simulink model "pendulum_on_a_cart_ctrld"  (R2021a)
settings: Solver=daessc  StartTime=0.0  StopTime=simlength  RelTol=1e-3
undefined symbols (not defined in the file): Ad, Aled, Bd, Bled, C, Cle, g, Ked, Ld, Lled, tc, ts
libraries: nesl_utility x14, fl_lib x8, pendulum_on_a_cart_lib x2
settings Model: SimulationMode=accelerator  Creator=dbagn  LastModifiedBy=dabagnara
settings SolverCC: AlgebraicLoopSolver=TrustRegion
settings DataIOCC: ReturnWorkspaceOutputs=off
settings DebuggingCC: SFMachineParentedDataDiag=warning

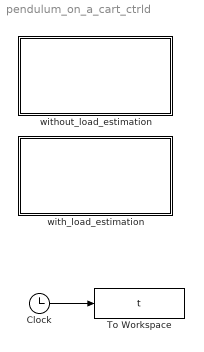
== system pendulum_on_a_cart_ctrld ==
  Clock : Clock
  To Workspace : ToWorkspace  VariableName=t  SampleTime=tc
      settings: MaxDataPoints=Nc
  with_load_estimation : Subsystem
  without_load_estimation : Subsystem
  wires:
  Clock/1 -> To Workspace/1

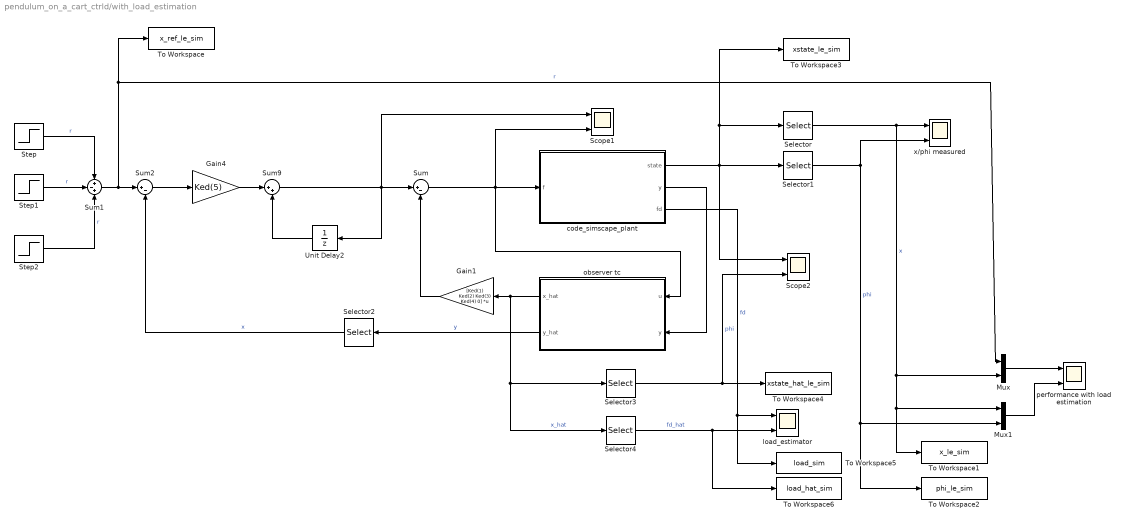
== system pendulum_on_a_cart_ctrld/with_load_estimation ==
  Gain1 : Gain  Gain=[Ked(1) Ked(2) Ked(3) Ked(4) 0]  Multiplication=Matrix(K*u)
  Gain4 : Gain  Gain=Ked(5)
  Mux : Mux  Inputs=2
  Mux1 : Mux  Inputs=2
  Scope1 : Scope  NumInputPorts=2
  Scope2 : Scope  NumInputPorts=2
  Selector : Selector  InputPortWidth=4  IndexOptions=Index vector (dialog)  Indices=1  OutputSizes=1
  Selector1 : Selector  InputPortWidth=4  IndexOptions=Index vector (dialog)  Indices=3  OutputSizes=1
  Selector2 : Selector  InputPortWidth=2  IndexOptions=Index vector (dialog)  Indices=1  OutputSizes=1
  Selector3 : Selector  InputPortWidth=5  IndexOptions=Index vector (dialog)  Indices=[1 2 3 4]  OutputSizes=1
  Selector4 : Selector  InputPortWidth=5  IndexOptions=Index vector (dialog)  Indices=5  OutputSizes=1
  Step : Step  SampleTime=0
  Step1 : Step  Time=8  After=2  SampleTime=0
  Step2 : Step  Time=25  SampleTime=0
  Sum : Sum  Inputs=|+-
  Sum1 : Sum  Inputs=+-+
  Sum2 : Sum  Inputs=|+-
  Sum9 : Sum  Inputs=|++
  To Workspace : ToWorkspace  VariableName=x_ref_le_sim  SampleTime=tc
      settings: MaxDataPoints=Nc
  To Workspace1 : ToWorkspace  VariableName=x_le_sim  SampleTime=tc
      settings: MaxDataPoints=Nc
  To Workspace2 : ToWorkspace  VariableName=phi_le_sim  SampleTime=tc
      settings: MaxDataPoints=Nc
  To Workspace3 : ToWorkspace  VariableName=xstate_le_sim  SampleTime=tc
      settings: MaxDataPoints=Nc
  To Workspace4 : ToWorkspace  VariableName=xstate_hat_le_sim  SampleTime=tc
      settings: MaxDataPoints=Nc
  To Workspace5 : ToWorkspace  VariableName=load_sim  SampleTime=tc
      settings: MaxDataPoints=Nc
  To Workspace6 : ToWorkspace  VariableName=load_hat_sim  SampleTime=tc
      settings: MaxDataPoints=Nc
  Unit Delay2 : UnitDelay  SampleTime=ts  HasFrameUpgradeWarning=on
  "code_simscape_plant " : Subsystem
  load_estimator : Scope  NumInputPorts=2
  observer tc : Subsystem
  performance with load estimation : Scope  NumInputPorts=2
  x/phi measured : Scope  NumInputPorts=2
  wires:
  Sum1/1 -> To Workspace/1, Mux/1, Sum2/1  "r"
  Sum2/1 -> Gain4/1
  Step1/1 -> Sum1/2  "r"
  Step/1 -> Sum1/1  "r"
  Gain4/1 -> Sum9/1
  observer tc/2(y_hat) -> Selector2/1  "y"
  Selector1/1 -> To Workspace2/1, Mux1/2, x/phi measured/2  "phi"
  "code_simscape_plant "/1(state) -> Scope2/1, Selector1/1, To Workspace3/1, Selector/1
  observer tc/1(x_hat) -> Gain1/1, Selector3/1, Selector4/1  "x_hat"
  Sum9/1 -> Scope1/1, Sum/1, Unit Delay2/1
  "code_simscape_plant "/2(y) -> observer tc/2(y)
  Selector2/1 -> Sum2/2  "x"
  Gain1/1 -> Sum/2
  Unit Delay2/1 -> Sum9/2
  Selector3/1 -> To Workspace4/1, Scope2/2  "phi"
  "code_simscape_plant "/3(fd) -> To Workspace5/1, load_estimator/1  "fd"
  Selector4/1 -> To Workspace6/1, load_estimator/2  "fd_hat"
  Step2/1 -> Sum1/3  "r"
  Mux1/1 -> performance with load estimation/2
  Mux/1 -> performance with load estimation/1
  Selector/1 -> To Workspace1/1, Mux1/1, Mux/2, x/phi measured/1  "x"
  Sum/1 -> observer tc/1(u), Scope1/2, "code_simscape_plant "/1(f)

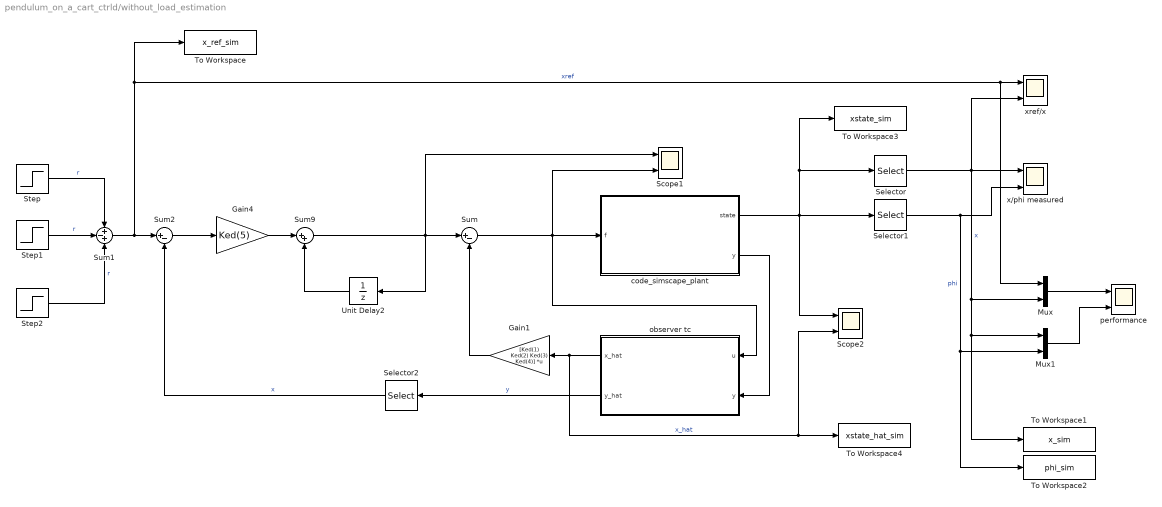
== system pendulum_on_a_cart_ctrld/without_load_estimation ==
  Gain1 : Gain  Gain=[Ked(1) Ked(2) Ked(3) Ked(4)]  Multiplication=Matrix(K*u)
  Gain4 : Gain  Gain=Ked(5)
  Mux : Mux  Inputs=2
  Mux1 : Mux  Inputs=2
  Scope1 : Scope  NumInputPorts=2
  Scope2 : Scope  NumInputPorts=2
  Selector : Selector  InputPortWidth=4  IndexOptions=Index vector (dialog)  Indices=1  OutputSizes=1
  Selector1 : Selector  InputPortWidth=4  IndexOptions=Index vector (dialog)  Indices=3  OutputSizes=1
  Selector2 : Selector  InputPortWidth=2  IndexOptions=Index vector (dialog)  Indices=1  OutputSizes=1
  Step : Step  SampleTime=0
  Step1 : Step  Time=8  After=2  SampleTime=0
  Step2 : Step  Time=25  SampleTime=0
  Sum : Sum  Inputs=|+-
  Sum1 : Sum  Inputs=+-+
  Sum2 : Sum  Inputs=|+-
  Sum9 : Sum  Inputs=|++
  To Workspace : ToWorkspace  VariableName=x_ref_sim  SampleTime=tc
      settings: MaxDataPoints=Nc
  To Workspace1 : ToWorkspace  VariableName=x_sim  SampleTime=tc
      settings: MaxDataPoints=Nc
  To Workspace2 : ToWorkspace  VariableName=phi_sim  SampleTime=tc
      settings: MaxDataPoints=Nc
  To Workspace3 : ToWorkspace  VariableName=xstate_sim  SampleTime=tc
      settings: MaxDataPoints=Nc
  To Workspace4 : ToWorkspace  VariableName=xstate_hat_sim  SampleTime=tc
      settings: MaxDataPoints=Nc
  Unit Delay2 : UnitDelay  SampleTime=ts  HasFrameUpgradeWarning=on
  "code_simscape_plant " : Subsystem
  observer tc : Subsystem
  performance : Scope  NumInputPorts=2
  x/phi measured : Scope  NumInputPorts=2
  xref/x : Scope  NumInputPorts=2
  wires:
  Unit Delay2/1 -> Sum9/2
  Gain1/1 -> Sum/2
  Selector2/1 -> Sum2/2  "x"
  Sum/1 -> "code_simscape_plant "/1(f), Scope1/2, observer tc/1(u)
  Selector/1 -> To Workspace1/1, Mux1/1, Mux/2, x/phi measured/1, xref/x/2  "x"
  "code_simscape_plant "/2(y) -> observer tc/2(y)
  Sum9/1 -> Unit Delay2/1, Sum/1, Scope1/1
  observer tc/1(x_hat) -> Scope2/2, To Workspace4/1, Gain1/1  "x_hat"
  "code_simscape_plant "/1(state) -> To Workspace3/1, Selector/1, Scope2/1, Selector1/1
  Selector1/1 -> To Workspace2/1, Mux1/2, x/phi measured/2  "phi"
  observer tc/2(y_hat) -> Selector2/1  "y"
  Gain4/1 -> Sum9/1
  Sum2/1 -> Gain4/1
  Sum1/1 -> To Workspace/1, Mux/1, xref/x/1, Sum2/1  "xref"
  Step/1 -> Sum1/1  "r"
  Step2/1 -> Sum1/3  "r"
  Step1/1 -> Sum1/2  "r"
  Mux/1 -> performance/1
  Mux1/1 -> performance/2

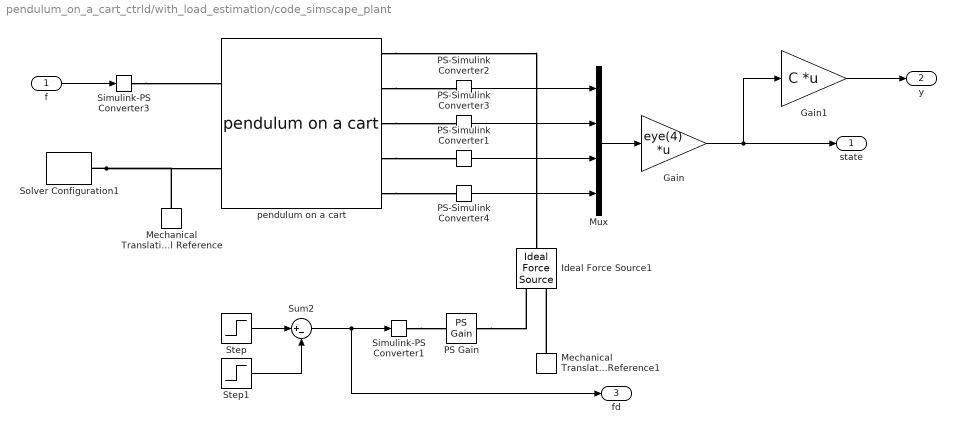
== system pendulum_on_a_cart_ctrld/with_load_estimation/code_simscape_plant  ==
  f : Inport
  Gain : Gain  Gain=eye(4)  Multiplication=Matrix(K*u)
  Gain1 : Gain  Gain=C  Multiplication=Matrix(K*u)
  Ideal Force Source1 : fl_lib/Mechanical/Mechanical Sources/Ideal Force Source
  Mechanical Translational Reference : fl_lib/Mechanical/Translational Elements/Mechanical Translational Reference
  Mechanical Translational Reference1 : fl_lib/Mechanical/Translational Elements/Mechanical Translational Reference
  Mux : Mux
  PS Gain : fl_lib/Physical Signals/Functions/PS Gain  gain=-1
  PS-Simulink Converter1 : nesl_utility/PS-Simulink Converter  PhysicalDomain=network_engine_domain  SubClassName=ps_output  LeftPortType=input  RightPortType=output  PseudoPeriodic=off  Frequencies=[]  Unit=rad  AffineConversion=on
      settings: SourceProductBaseCode=PW,SS
  PS-Simulink Converter2 : nesl_utility/PS-Simulink Converter  PhysicalDomain=network_engine_domain  SubClassName=ps_output  LeftPortType=input  RightPortType=output  PseudoPeriodic=off  Frequencies=[]  Unit=m  AffineConversion=on
      settings: SourceProductBaseCode=PW,SS
  PS-Simulink Converter3 : nesl_utility/PS-Simulink Converter  PhysicalDomain=network_engine_domain  SubClassName=ps_output  LeftPortType=input  RightPortType=output  PseudoPeriodic=off  Frequencies=[]  Unit=m/s  AffineConversion=on
      settings: SourceProductBaseCode=PW,SS
  PS-Simulink Converter4 : nesl_utility/PS-Simulink Converter  PhysicalDomain=network_engine_domain  SubClassName=ps_output  LeftPortType=input  RightPortType=output  PseudoPeriodic=off  Frequencies=[]  Unit=rad/s  AffineConversion=on
      settings: SourceProductBaseCode=PW,SS
  Simulink-PS Converter1 : nesl_utility/Simulink-PS Converter  PhysicalDomain=network_engine_domain  SubClassName=ps_input  LeftPortType=input  RightPortType=output  PseudoPeriodic=off  Frequencies=[]  NoiseDistribution=none  NoiseParameters=[]  Unit=N  AffineConversion=off  FilteringAndDerivatives=provide  SimscapeFilterOrder=1  InputFilterTimeConstant=0.001  UdotUserProvided=0
      settings: SourceProductBaseCode=PW,SS
  Simulink-PS Converter3 : nesl_utility/Simulink-PS Converter  PhysicalDomain=network_engine_domain  SubClassName=ps_input  LeftPortType=input  RightPortType=output  PseudoPeriodic=off  Frequencies=[]  NoiseDistribution=none  NoiseParameters=[]  Unit=N  AffineConversion=off  FilteringAndDerivatives=provide  SimscapeFilterOrder=1  InputFilterTimeConstant=0.001  UdotUserProvided=0
      settings: SourceProductBaseCode=PW,SS
  Solver Configuration1 : nesl_utility/Solver Configuration  PhysicalDomain=network_engine_domain  SubClassName=solver  LeftPortType=input  RightPortType=generic  Tones=[]  Harmonics=[]  SimulateNoise=off  Profile=off  UseLocalSampling=off  EnableSwitchedLinearOptims=on  FrequencyDomain=off  UseCCode=off  RelTol=0.001  AbsTol=1e-06  MinStep=1e-09  ToWorkspace=off  RevertToSquareIcSolve=off  NumHomotopyIterations=100  PhasorMode=off  PhasorModeNumHarmonics=1  DoDC=on  ResidualTolerance=1e-09  UseLocalSolver=off  LocalSolverChoice=NE_BACKWARD_EULER_ADVANCER  LocalSolverSampleTime=ts  DoFixedCost=off  MaxNonlinIter=3  MaxModeIter=2  ComputeImpulses=off  ImpulseIterations=2  LinearAlgebra=auto  EquationFormulation=NE_TIME_EF  DelaysMemoryBudget=1024  AutomaticFiltering=on  FilteringTimeConstant=0.001  PartitionStorageMethod=AS_NEEDED  PartitionMemoryBudget=1024  PartitionMethod=ROBUST
      settings: SourceProductBaseCode=PW,SS
  Step : Step  Time=17.5  After=1000  SampleTime=0
  Step1 : Step  Time=30  After=1000  SampleTime=0
  Sum2 : Sum  Inputs=|+-
  pendulum on a cart : pendulum_on_a_cart_lib/pendulum on a cart  m0=m0 kg  m1=m1 kg  J1=J1 kg*m^2  s1=s1 m  b0=b0 N/(m/s)  b1=b1 N*m/(rad/s)  g=g m/s^2  d_specify=off  d_priority=None  d=0 N  d_nominal_specify=off  d_nominal_unit=N  d_nominal_value=1  x1_specify=off  x1_priority=High  x1=0 m  x1_nominal_specify=off  x1_nominal_unit=m  x1_nominal_value=1  x2_specify=off  x2_priority=High  x2=0 m/s  x2_nominal_specify=off  x2_nominal_unit=m/s  x2_nominal_value=1  x3_specify=off  x3_priority=High  x3=pi rad  x3_nominal_specify=off  x3_nominal_unit=rad  x3_nominal_value=1  x4_specify=off  x4_priority=High  x4=0 rad/s  x4_nominal_specify=off  x4_nominal_unit=rad/s  x4_nominal_value=1
      settings: InternalSimscapePortConfiguration="{\"Bottom\":[],\"Left\":[{\"id\":\"f\",\"label\":\"f\",\"type\":\"input\"},{\"id\":\"P1\",\"label\":\"P1\",\"type\":\"foundation.mechanical.translational.translational\"}],\"Right\":[{\"id\":\"P2\",\"label\":\"P2\",\"type\":\"foundation.mechanical.translational.translational\"},{\"id\":\"x\",\"label\":\"x\",\"type\":\"output\"},{\"id\":\"v\",\"label\":\"v\",\"type\":\"output\"},{\"id\":\"phi\",\"label\":\"phi\",\"type\":\"output\"},{\"id\":\"omega\",\"label\":\"omega\",\"type\":\"output\"}],\"Top\":[]}"
  state : Outport
  y : Outport  Port=2
  fd : Outport  Port=3
  wires:
  Sum2/1 -> fd/1, Simulink-PS Converter1/1
  Gain1/1 -> y/1
  Gain/1 -> state/1, Gain1/1
  Mux/1 -> Gain/1
  PS-Simulink Converter4/1 -> Mux/4
  PS-Simulink Converter1/1 -> Mux/3
  f/1 -> Simulink-PS Converter3/1
  PS-Simulink Converter3/1 -> Mux/2
  PS-Simulink Converter2/1 -> Mux/1
  Step1/1 -> Sum2/2
  Step/1 -> Sum2/1
  connections:
  Simulink-PS Converter3/RConn1 -- pendulum on a cart/LConn1
  Mechanical Translational Reference1/LConn1 -- Ideal Force Source1/RConn2
  pendulum on a cart/RConn1 -- Ideal Force Source1/LConn1
  Solver Configuration1/RConn1 -- pendulum on a cart/LConn2 -- Mechanical Translational Reference/LConn1
  pendulum on a cart/RConn2 -- PS-Simulink Converter2/LConn1
  pendulum on a cart/RConn3 -- PS-Simulink Converter3/LConn1
  pendulum on a cart/RConn4 -- PS-Simulink Converter1/LConn1
  pendulum on a cart/RConn5 -- PS-Simulink Converter4/LConn1
  Simulink-PS Converter1/RConn1 -- PS Gain/LConn1
  PS Gain/RConn1 -- Ideal Force Source1/RConn1

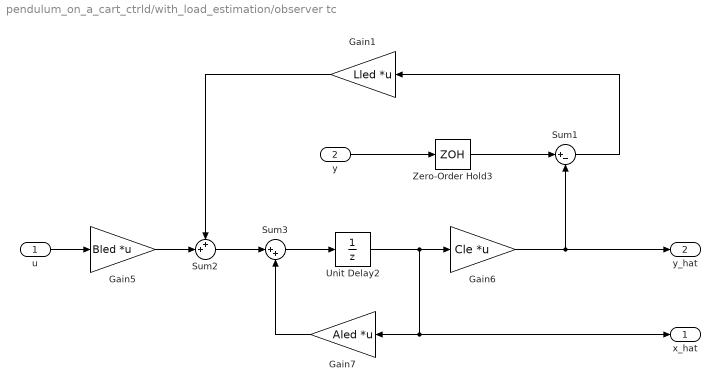
== system pendulum_on_a_cart_ctrld/with_load_estimation/observer tc ==
  u : Inport
  y : Inport  Port=2
  Gain1 : Gain  Gain=Lled  Multiplication=Matrix(K*u)
  Gain5 : Gain  Gain=Bled  Multiplication=Matrix(K*u)
  Gain6 : Gain  Gain=Cle  Multiplication=Matrix(K*u)
  Gain7 : Gain  Gain=Aled  Multiplication=Matrix(K*u)
  Sum1 : Sum  Inputs=|+-
  Sum2 : Sum  Inputs=++|
  Sum3 : Sum  Inputs=|++
  Unit Delay2 : UnitDelay  SampleTime=ts  HasFrameUpgradeWarning=on
  Zero-Order Hold3 : ZeroOrderHold  SampleTime=ts
  x_hat : Outport
  y_hat : Outport  Port=2
  wires:
  Unit Delay2/1 -> Gain6/1, Gain7/1, x_hat/1
  Zero-Order Hold3/1 -> Sum1/1
  y/1 -> Zero-Order Hold3/1
  Gain5/1 -> Sum2/2
  Gain1/1 -> Sum2/1
  u/1 -> Gain5/1
  Sum1/1 -> Gain1/1
  Gain6/1 -> Sum1/2, y_hat/1
  Gain7/1 -> Sum3/2
  Sum3/1 -> Unit Delay2/1
  Sum2/1 -> Sum3/1

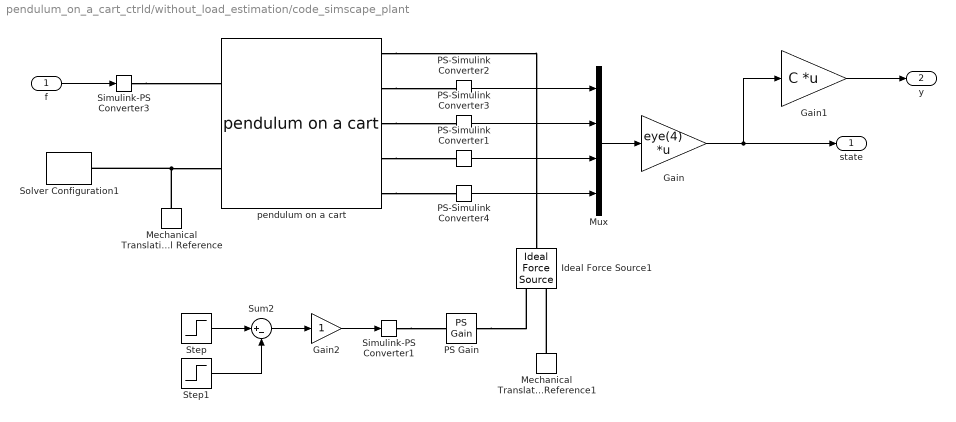
== system pendulum_on_a_cart_ctrld/without_load_estimation/code_simscape_plant  ==
  f : Inport
  Gain : Gain  Gain=eye(4)  Multiplication=Matrix(K*u)
  Gain1 : Gain  Gain=C  Multiplication=Matrix(K*u)
  Gain2 : Gain
  Ideal Force Source1 : fl_lib/Mechanical/Mechanical Sources/Ideal Force Source
  Mechanical Translational Reference : fl_lib/Mechanical/Translational Elements/Mechanical Translational Reference
  Mechanical Translational Reference1 : fl_lib/Mechanical/Translational Elements/Mechanical Translational Reference
  Mux : Mux
  PS Gain : fl_lib/Physical Signals/Functions/PS Gain  gain=-1
  PS-Simulink Converter1 : nesl_utility/PS-Simulink Converter  PhysicalDomain=network_engine_domain  SubClassName=ps_output  LeftPortType=input  RightPortType=output  PseudoPeriodic=off  Frequencies=[]  Unit=rad  AffineConversion=on
      settings: SourceProductBaseCode=PW,SS
  PS-Simulink Converter2 : nesl_utility/PS-Simulink Converter  PhysicalDomain=network_engine_domain  SubClassName=ps_output  LeftPortType=input  RightPortType=output  PseudoPeriodic=off  Frequencies=[]  Unit=m  AffineConversion=on
      settings: SourceProductBaseCode=PW,SS
  PS-Simulink Converter3 : nesl_utility/PS-Simulink Converter  PhysicalDomain=network_engine_domain  SubClassName=ps_output  LeftPortType=input  RightPortType=output  PseudoPeriodic=off  Frequencies=[]  Unit=m/s  AffineConversion=on
      settings: SourceProductBaseCode=PW,SS
  PS-Simulink Converter4 : nesl_utility/PS-Simulink Converter  PhysicalDomain=network_engine_domain  SubClassName=ps_output  LeftPortType=input  RightPortType=output  PseudoPeriodic=off  Frequencies=[]  Unit=rad/s  AffineConversion=on
      settings: SourceProductBaseCode=PW,SS
  Simulink-PS Converter1 : nesl_utility/Simulink-PS Converter  PhysicalDomain=network_engine_domain  SubClassName=ps_input  LeftPortType=input  RightPortType=output  PseudoPeriodic=off  Frequencies=[]  NoiseDistribution=none  NoiseParameters=[]  Unit=N  AffineConversion=off  FilteringAndDerivatives=provide  SimscapeFilterOrder=1  InputFilterTimeConstant=0.001  UdotUserProvided=0
      settings: SourceProductBaseCode=PW,SS
  Simulink-PS Converter3 : nesl_utility/Simulink-PS Converter  PhysicalDomain=network_engine_domain  SubClassName=ps_input  LeftPortType=input  RightPortType=output  PseudoPeriodic=off  Frequencies=[]  NoiseDistribution=none  NoiseParameters=[]  Unit=N  AffineConversion=off  FilteringAndDerivatives=provide  SimscapeFilterOrder=1  InputFilterTimeConstant=0.001  UdotUserProvided=0
      settings: SourceProductBaseCode=PW,SS
  Solver Configuration1 : nesl_utility/Solver Configuration  PhysicalDomain=network_engine_domain  SubClassName=solver  LeftPortType=input  RightPortType=generic  Tones=[]  Harmonics=[]  SimulateNoise=off  Profile=off  UseLocalSampling=off  EnableSwitchedLinearOptims=on  FrequencyDomain=off  UseCCode=off  RelTol=0.001  AbsTol=1e-06  MinStep=1e-09  ToWorkspace=off  RevertToSquareIcSolve=off  NumHomotopyIterations=100  PhasorMode=off  PhasorModeNumHarmonics=1  DoDC=on  ResidualTolerance=1e-09  UseLocalSolver=off  LocalSolverChoice=NE_BACKWARD_EULER_ADVANCER  LocalSolverSampleTime=ts  DoFixedCost=off  MaxNonlinIter=3  MaxModeIter=2  ComputeImpulses=off  ImpulseIterations=2  LinearAlgebra=auto  EquationFormulation=NE_TIME_EF  DelaysMemoryBudget=1024  AutomaticFiltering=on  FilteringTimeConstant=0.001  PartitionStorageMethod=AS_NEEDED  PartitionMemoryBudget=1024  PartitionMethod=ROBUST
      settings: SourceProductBaseCode=PW,SS
  Step : Step  Time=17.5  After=1000  SampleTime=0
  Step1 : Step  Time=30  After=1000  SampleTime=0
  Sum2 : Sum  Inputs=|+-
  pendulum on a cart : pendulum_on_a_cart_lib/pendulum on a cart  m0=m0 kg  m1=m1 kg  J1=J1 kg*m^2  s1=s1 m  b0=b0 N/(m/s)  b1=b1 N*m/(rad/s)  g=g m/s^2  d_specify=off  d_priority=None  d=0 N  d_nominal_specify=off  d_nominal_unit=N  d_nominal_value=1  x1_specify=off  x1_priority=High  x1=0 m  x1_nominal_specify=off  x1_nominal_unit=m  x1_nominal_value=1  x2_specify=off  x2_priority=High  x2=0 m/s  x2_nominal_specify=off  x2_nominal_unit=m/s  x2_nominal_value=1  x3_specify=off  x3_priority=High  x3=pi rad  x3_nominal_specify=off  x3_nominal_unit=rad  x3_nominal_value=1  x4_specify=off  x4_priority=High  x4=0 rad/s  x4_nominal_specify=off  x4_nominal_unit=rad/s  x4_nominal_value=1
      settings: InternalSimscapePortConfiguration="{\"Bottom\":[],\"Left\":[{\"id\":\"f\",\"label\":\"f\",\"type\":\"input\"},{\"id\":\"P1\",\"label\":\"P1\",\"type\":\"foundation.mechanical.translational.translational\"}],\"Right\":[{\"id\":\"P2\",\"label\":\"P2\",\"type\":\"foundation.mechanical.translational.translational\"},{\"id\":\"x\",\"label\":\"x\",\"type\":\"output\"},{\"id\":\"v\",\"label\":\"v\",\"type\":\"output\"},{\"id\":\"phi\",\"label\":\"phi\",\"type\":\"output\"},{\"id\":\"omega\",\"label\":\"omega\",\"type\":\"output\"}],\"Top\":[]}"
  state : Outport
  y : Outport  Port=2
  wires:
  PS-Simulink Converter2/1 -> Mux/1
  PS-Simulink Converter3/1 -> Mux/2
  f/1 -> Simulink-PS Converter3/1
  PS-Simulink Converter1/1 -> Mux/3
  PS-Simulink Converter4/1 -> Mux/4
  Mux/1 -> Gain/1
  Gain/1 -> Gain1/1, state/1
  Gain1/1 -> y/1
  Step/1 -> Sum2/1
  Sum2/1 -> Gain2/1
  Step1/1 -> Sum2/2
  Gain2/1 -> Simulink-PS Converter1/1
  connections:
  pendulum on a cart/RConn5 -- PS-Simulink Converter4/LConn1
  pendulum on a cart/RConn4 -- PS-Simulink Converter1/LConn1
  pendulum on a cart/RConn3 -- PS-Simulink Converter3/LConn1
  pendulum on a cart/RConn2 -- PS-Simulink Converter2/LConn1
  Mechanical Translational Reference/LConn1 -- pendulum on a cart/LConn2 -- Solver Configuration1/RConn1
  pendulum on a cart/RConn1 -- Ideal Force Source1/LConn1
  Mechanical Translational Reference1/LConn1 -- Ideal Force Source1/RConn2
  Simulink-PS Converter3/RConn1 -- pendulum on a cart/LConn1
  Simulink-PS Converter1/RConn1 -- PS Gain/LConn1
  PS Gain/RConn1 -- Ideal Force Source1/RConn1

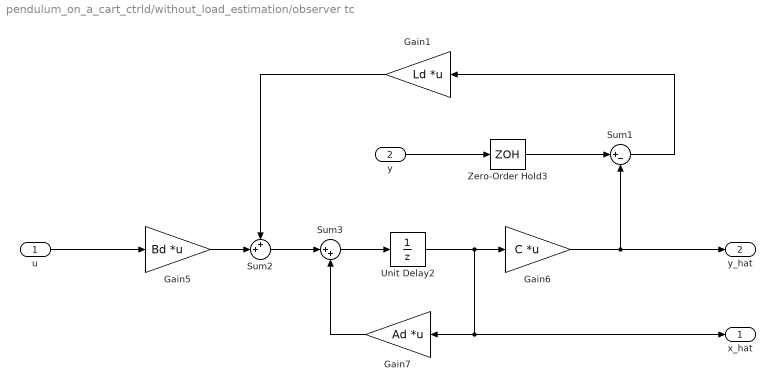
== system pendulum_on_a_cart_ctrld/without_load_estimation/observer tc ==
  u : Inport
  y : Inport  Port=2
  Gain1 : Gain  Gain=Ld  Multiplication=Matrix(K*u)
  Gain5 : Gain  Gain=Bd  Multiplication=Matrix(K*u)
  Gain6 : Gain  Gain=C  Multiplication=Matrix(K*u)
  Gain7 : Gain  Gain=Ad  Multiplication=Matrix(K*u)
  Sum1 : Sum  Inputs=|+-
  Sum2 : Sum  Inputs=++|
  Sum3 : Sum  Inputs=|++
  Unit Delay2 : UnitDelay  SampleTime=ts  HasFrameUpgradeWarning=on
  Zero-Order Hold3 : ZeroOrderHold  SampleTime=ts
  x_hat : Outport
  y_hat : Outport  Port=2
  wires:
  Sum2/1 -> Sum3/1
  Sum3/1 -> Unit Delay2/1
  Gain7/1 -> Sum3/2
  Gain6/1 -> y_hat/1, Sum1/2
  Sum1/1 -> Gain1/1
  u/1 -> Gain5/1
  Gain1/1 -> Sum2/1
  Gain5/1 -> Sum2/2
  y/1 -> Zero-Order Hold3/1
  Zero-Order Hold3/1 -> Sum1/1
  Unit Delay2/1 -> x_hat/1, Gain7/1, Gain6/1
